simulink model "ControlSystemProject"  (R2023a)
settings: Solver=VariableStepAuto  StartTime=0.0  StopTime=100  RelTol=1e-3
settings Model: Creator=mazen  LastModifiedBy=mazen

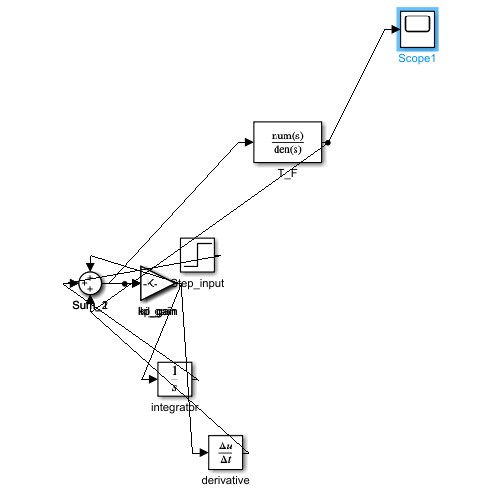
[thumbnail: Simulink's stored preview of the top-level diagram]
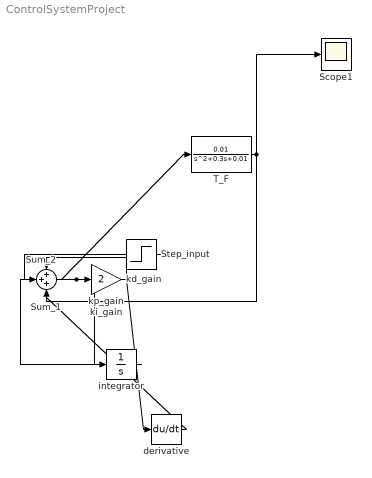
== system ControlSystemProject ==
  Scope1 : Scope
  Step_input : Step  SampleTime=0
  Sum_1 : Sum  Inputs=|+-
  Sum_2 : Sum  Inputs=+++
  T_F : TransferFcn  Numerator=[0.01]  Denominator=[1 0.3 0.01]
  derivative : Derivative
  integrator : Integrator
  kd_gain : Gain  Gain=1e-9
  ki_gain : Gain  Gain=0.1
  kp_gain : Gain  Gain=2
  wires:
  Step_input/1 -> Sum_1/1
  Sum_1/1 -> kp_gain/1, ki_gain/1, kd_gain/1
  kp_gain/1 -> Sum_2/1
  ki_gain/1 -> integrator/1
  kd_gain/1 -> derivative/1
  integrator/1 -> Sum_2/2
  derivative/1 -> Sum_2/3
  Sum_2/1 -> T_F/1
  T_F/1 -> Sum_1/2, Scope1/1
